simulink model "cascaded_droop_vi"  (R2021b)
settings: Solver=ode23t  StartTime=0.0  StopTime=20  RelTol=1e-3
values from neighbouring files (symbols this model uses):
  Cf_1 = 16e-6    (= 1.6e-05)    [parameters.m]
  fn = 50    [parameters.m]
  G_int = c2d(tf([wv 0],[1 wv]),Ts/2,'tustin')    [parameters.m]
  G_LPFd2 = c2d(tf([k*wn 0],[1 k*wn wn^2]),Ts/2,'tustin')    [parameters.m]
  Ilim = In    [parameters.m]
  ki_u = kp_u/Ti_u    [parameters.m]
  Kic_1 = (Rf_1)/T_i    (= 640)    [parameters.m]
  kp = delta_f/delta_P    (= 0.002)    [parameters.m]
  kp_u = Cf*w_c    [parameters.m]
  Kpc_1 = Rf_1/(exp(Rf_1/Lf_1*Ts/2)-1)    [parameters.m]
  Lf_1 = 5.6e-3    (= 0.0056)    [parameters.m]
  Lg_1 = 1e-3    (= 0.001)    [parameters.m]
  Lv = kQ/wn    [parameters.m]
  Pr = 2000    [parameters.m]
  RCf_1 = 0    [parameters.m]
  Rf_1 = 0.1    [parameters.m]
  Rg_1 = 0.08    [parameters.m]
  Rv = kQ/10    [parameters.m]
  Ts = 1/fs    (= 0.0003125)    [parameters.m]
  Ts_sim = Ts/100    (= 3.125e-06)    [parameters.m]
  Vdc = 800*sf_v    [parameters.m]
  Vn = 181*sqrt(2)*sf_v    [parameters.m]
  wn = 2*pi*fn    (= 314.159265359)    [parameters.m]
undefined symbols (not defined in the file or in its folder): DiscIntNeverNeededParam, plecs
libraries: spsVoltageMeasurementLib x15, spsCurrentMeasurementLib x12, spsabctoAlphaBetaZeroLib x10, spsThreePhaseSeriesRLCBranchLib x8, eeGeneralControl x7, spsThreePhaseVIMeasurementLib x4, spsGroundLib x3, spsThreePhaseSourceLib x2, spsDCVoltageSourceLib x2, spsEdgeDetectorLib x2, spsTriangleGeneratorLib x2, spsThreePhaseBreakerLib x2
(part 2 of 2)

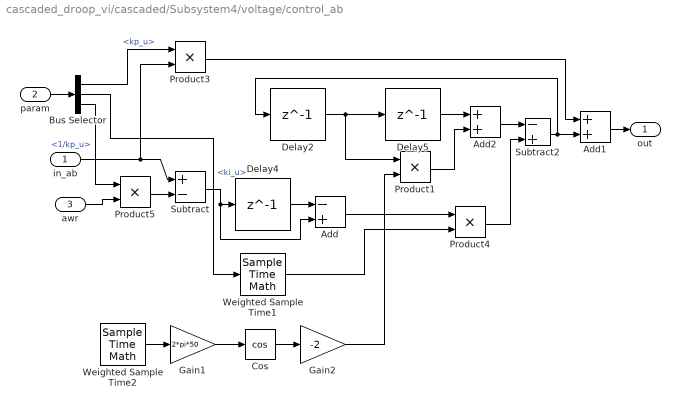
== system cascaded_droop_vi/cascaded/Subsystem4/voltage/control_ab ==
  in_ab : Inport
  param : Inport  Port=2
  awr : Inport  Port=3
  Add : Sum  Inputs=-+  AccumDataTypeStr=single
  Add1 : Sum
  Add2 : Sum
  Bus Selector : BusSelector  OutputSignals=kp_u,ki_u,1/kp_u
  Cos : Trigonometry  Operator=cos
  Delay2 : Delay  DelayLength=1  InitialCondition=0
  Delay4 : Delay  DelayLength=1  InitialCondition=0
  Delay5 : Delay  DelayLength=1  InitialCondition=0
  Gain1 : Gain  Gain=2*pi*50
  Gain2 : Gain  Gain=-2
  Product{1,3..5} (4 alike) : Product
  Subtract : Sum  Inputs=+-
  Subtract2 : Sum  Inputs=-+
  Weighted Sample Time1 : SampleTimeMath  TsampMathOp=*
  Weighted Sample Time2 : SampleTimeMath  TsampMathOp=Ts Only
  out : Outport  VectorParamsAs1DForOutWhenUnconnected=off
  wires:
  Gain2/1 -> Product1/2
  Cos/1 -> Gain2/1
  Gain1/1 -> Cos/1
  Weighted Sample Time2/1 -> Gain1/1
  Bus Selector/3 -> Product5/1  "<1/kp_u>"
  awr/1 -> Product5/2
  Product5/1 -> Subtract/2
  Weighted Sample Time1/1 -> Product4/2
  Bus Selector/2 -> Weighted Sample Time1/1  "<ki_u>"
  Bus Selector/1 -> Product3/1  "<kp_u>"
  Product3/1 -> Add1/1
  Add2/1 -> Subtract2/1
  Delay2/1 -> Delay5/1, Product1/1
  Subtract2/1 -> Add1/2, Delay2/1
  Delay5/1 -> Add2/1
  in_ab/1 -> Subtract/1, Product3/2
  Add/1 -> Product4/1
  Subtract/1 -> Add/2, Delay4/1
  Delay4/1 -> Add/1
  Product4/1 -> Subtract2/2
  Add1/1 -> out/1
  Product1/1 -> Add2/2
  param/1 -> Bus Selector/1

== system cascaded_droop_vi/cascaded/Subsystem4/voltage/current_FF ==
  a : Inport
  b : Inport  Port=2
  g_FF : Inport  Port=3
  Add5 : Sum
  Product : Product
  ab_out : Outport  VectorParamsAs1DForOutWhenUnconnected=off
  wires:
  Add5/1 -> ab_out/1
  a/1 -> Add5/1
  g_FF/1 -> Product/2
  b/1 -> Product/1
  Product/1 -> Add5/2

== system cascaded_droop_vi/cascaded controller/cascaded/Cascaded Loop/THI1 ==
  THI gain : Inport
  abc : Inport  Port=2
  ab : Inport  Port=3
  Add : Sum  Inputs=+++
  Add{1..4} (4 alike) : Sum
  Demux : Demux  Outputs=3
  Demux1 : Demux  Outputs=2
  Divide : Product  Inputs=*/*
  Fcn : Fcn  Expr=u^3
  Fcn1 : Fcn  Expr=u^3
  Fcn2 : Fcn  Expr=u^3
  Mux : Mux  Inputs=3
  Square : Math  Operator=square  SignedPower=on  RndMeth=Zero  SaturateOnIntegerOverflow=on
  Square1 : Math  Operator=square  SignedPower=on  RndMeth=Zero  SaturateOnIntegerOverflow=on
  abc_out : Outport  VectorParamsAs1DForOutWhenUnconnected=off
  wires:
  Demux/2 -> Add3/1, Fcn1/1
  Fcn2/1 -> Add/3
  Fcn1/1 -> Add/2
  Fcn/1 -> Add/1
  Mux/1 -> abc_out/1
  Add4/1 -> Mux/3
  Add2/1 -> Mux/1
  Add3/1 -> Mux/2
  Divide/1 -> Add4/2, Add3/2, Add2/2
  THI gain/1 -> Divide/3
  Add1/1 -> Divide/2
  Add/1 -> Divide/1
  Square1/1 -> Add1/2
  Square/1 -> Add1/1
  Demux1/2 -> Square1/1
  Demux1/1 -> Square/1
  ab/1 -> Demux1/1
  Demux/1 -> Fcn/1, Add2/1
  Demux/3 -> Add4/1, Fcn2/1
  abc/1 -> Demux/1

== system cascaded_droop_vi/cascaded controller/cascaded/Cascaded Loop/Virtual impedance ==
  Ig_ab : Inport
  Discrete Transfer Fcn2 : DiscreteTransferFcn  Numerator=G_int.num{1}  Denominator=G_int.den{1}
  Gain1 : Gain  Gain=Rv
  Gain2 : Gain  Gain=Lv
  Sum3 : Sum  Inputs=|++
  U_Lv_ab : Outport  VectorParamsAs1DForOutWhenUnconnected=off
  wires:
  Sum3/1 -> U_Lv_ab/1
  Gain1/1 -> Sum3/2
  Gain2/1 -> Sum3/1
  Ig_ab/1 -> Discrete Transfer Fcn2/1, Gain1/1
  Discrete Transfer Fcn2/1 -> Gain2/1

== system cascaded_droop_vi/cascaded controller/cascaded/Cascaded Loop/current ==
  param : Inport
  I_ab_ref : Inport  Port=2
  I_ab : Inport  Port=3
  U_ab : Inport  Port=4
  Udc : Inport  Port=5
  Bus Selector : BusSelector  OutputSignals=E1,g_ff_v
  Delay : Delay  DelayLength=1  InitialCondition=0
  Discrete Transfer Fcn : DiscreteTransferFcn  Numerator=G_LPFd2.num{1}  Denominator=G_LPFd2.den{1}
  Divide : Product  Inputs=*/
  Gain : Gain  Gain=1/2
  Subtract : Sum  Inputs=+-
  Subtract1 : Sum  Inputs=+-
  Voltage_lim : Subsystem
  control_ab : Subsystem
  voltage_FF : Subsystem
  U_ab_inv : Outport  VectorParamsAs1DForOutWhenUnconnected=off
  wires:
  Discrete Transfer Fcn/1 -> voltage_FF/2(b)
  voltage_FF/1(ab_out) -> Voltage_lim/1(ab_in), Subtract/1
  Delay/1 -> control_ab/3(awr)
  Gain/1 -> Divide/2
  Divide/1 -> U_ab_inv/1
  Udc/1 -> Voltage_lim/2(Vdc), Gain/1
  U_ab/1 -> Discrete Transfer Fcn/1
  Subtract/1 -> Delay/1
  Bus Selector/2 -> voltage_FF/3(g_FF)  "<g_ff_v>"
  I_ab/1 -> Subtract1/2
  Subtract1/1 -> control_ab/1(in_ab)
  control_ab/1(out) -> voltage_FF/1(a)
  param/1 -> control_ab/2(param), Bus Selector/1
  I_ab_ref/1 -> Subtract1/1
  Voltage_lim/1(ab_out) -> Subtract/2, Divide/1

== system cascaded_droop_vi/cascaded controller/cascaded/Cascaded Loop/voltage ==
  param : Inport
  U_ab_ref : Inport  Port=2
  U_ab : Inport  Port=3
  Ig_ab : Inport  Port=4
  Bus Selector : BusSelector  OutputSignals=g_ff_i,Isat
  Current_lim : Subsystem
  Delay : Delay  DelayLength=1  InitialCondition=0
  Subtract : Sum  Inputs=+-
  Subtract1 : Sum  Inputs=+-
  control_ab : Subsystem
  current_FF : Subsystem
  I_ab_ref : Outport  VectorParamsAs1DForOutWhenUnconnected=off
  wires:
  Bus Selector/2 -> Current_lim/2(Isat)  "<Isat>"
  U_ab_ref/1 -> Subtract1/1
  param/1 -> Bus Selector/1, control_ab/2(param)
  control_ab/1(out) -> current_FF/1(a)
  Subtract1/1 -> control_ab/1(in_ab)
  U_ab/1 -> Subtract1/2
  Bus Selector/1 -> current_FF/3(g_FF)  "<g_ff_i>"
  Subtract/1 -> Delay/1
  Ig_ab/1 -> current_FF/2(b)
  Current_lim/1(ab_out) -> I_ab_ref/1, Subtract/2
  Delay/1 -> control_ab/3(awr)
  current_FF/1(ab_out) -> Subtract/1, Current_lim/1(ab_in)

== system cascaded_droop_vi/cascaded controller/cascaded/power calculation grid side/abc to alpha-beta3 ==
  abc : Inport
  Demux : Demux  Outputs=3
  Terminator1 : Terminator
  abc to Alpha-Beta-Zero : spsabctoAlphaBetaZeroLib/abc to Alpha-Beta-Zero
  alpha : Outport
  beta : Outport  Port=2
  wires:
  abc to Alpha-Beta-Zero/1 -> Demux/1
  abc/1 -> abc to Alpha-Beta-Zero/1
  Demux/3 -> Terminator1/1
  Demux/2 -> beta/1
  Demux/1 -> alpha/1

== system cascaded_droop_vi/cascaded/Subsystem4/current/Voltage_lim/Subsystem ==
  a : Inport
  b : Inport  Port=2
  Relational Operator : RelationalOperator  Operator=>  OutDataTypeStr=boolean  RndMeth=Simplest
  Switch : Switch  Criteria=u2 > Threshold  Threshold=0.5
  max : Outport  VectorParamsAs1DForOutWhenUnconnected=off
  wires:
  a/1 -> Relational Operator/1, Switch/1
  Switch/1 -> max/1
  b/1 -> Relational Operator/2, Switch/3
  Relational Operator/1 -> Switch/2

== system cascaded_droop_vi/cascaded/Subsystem4/current/Voltage_lim/pythagoras ==
  ab : Inport
  Sqrt : Sqrt  SaturateOnIntegerOverflow=on
  Square : Math  Operator=square  SignedPower=on  RndMeth=Zero  SaturateOnIntegerOverflow=on
  Sum of Elements : Sum  Inputs=+
  |ab| : Outport  VectorParamsAs1DForOutWhenUnconnected=off
  wires:
  Sum of Elements/1 -> Sqrt/1
  ab/1 -> Square/1
  Square/1 -> Sum of Elements/1
  Sqrt/1 -> |ab|/1

== system cascaded_droop_vi/cascaded/Subsystem4/voltage/Current_lim/Subsystem ==
  a : Inport
  b : Inport  Port=2
  Relational Operator : RelationalOperator  Operator=>  OutDataTypeStr=boolean  RndMeth=Simplest
  Switch : Switch  Criteria=u2 > Threshold  Threshold=0.5
  max : Outport  VectorParamsAs1DForOutWhenUnconnected=off
  wires:
  Relational Operator/1 -> Switch/2
  b/1 -> Switch/3, Relational Operator/2
  Switch/1 -> max/1
  a/1 -> Switch/1, Relational Operator/1

== system cascaded_droop_vi/cascaded/Subsystem4/voltage/Current_lim/pythagoras ==
  ab : Inport
  Sqrt : Sqrt  SaturateOnIntegerOverflow=on
  Square : Math  Operator=square  SignedPower=on  RndMeth=Zero  SaturateOnIntegerOverflow=on
  Sum of Elements : Sum  Inputs=+
  |ab| : Outport  VectorParamsAs1DForOutWhenUnconnected=off
  wires:
  Sqrt/1 -> |ab|/1
  Square/1 -> Sum of Elements/1
  ab/1 -> Square/1
  Sum of Elements/1 -> Sqrt/1

== system cascaded_droop_vi/cascaded controller/cascaded/Cascaded Loop/current/Voltage_lim ==
  ab_in : Inport
  Vdc : Inport  Port=2
  Divide : Product  Inputs=*/
  Divide1 : Product  Inputs=**
  Gain : Gain  Gain=1/sqrt(3)
  Subsystem : Subsystem
  pythagoras : Subsystem
  ab_out : Outport  VectorParamsAs1DForOutWhenUnconnected=off
  wires:
  Gain/1 -> Divide/1, Subsystem/2(b)
  ab_in/1 -> Divide1/2, pythagoras/1(ab)
  pythagoras/1(|ab|) -> Subsystem/1(a)
  Vdc/1 -> Gain/1
  Subsystem/1(max) -> Divide/2
  Divide/1 -> Divide1/1
  Divide1/1 -> ab_out/1

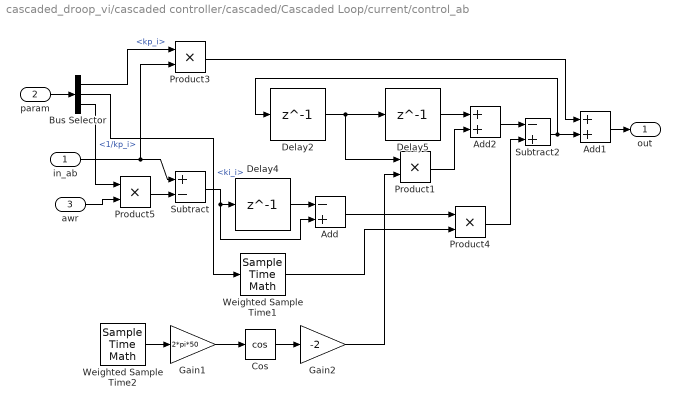
== system cascaded_droop_vi/cascaded controller/cascaded/Cascaded Loop/current/control_ab ==
  in_ab : Inport
  param : Inport  Port=2
  awr : Inport  Port=3
  Add : Sum  Inputs=-+  AccumDataTypeStr=single
  Add1 : Sum
  Add2 : Sum
  Bus Selector : BusSelector  OutputSignals=kp_i,ki_i,1/kp_i
  Cos : Trigonometry  Operator=cos
  Delay2 : Delay  DelayLength=1  InitialCondition=0
  Delay4 : Delay  DelayLength=1  InitialCondition=0
  Delay5 : Delay  DelayLength=1  InitialCondition=0
  Gain1 : Gain  Gain=2*pi*50
  Gain2 : Gain  Gain=-2
  Product{1,3..5} (4 alike) : Product
  Subtract : Sum  Inputs=+-
  Subtract2 : Sum  Inputs=-+
  Weighted Sample Time1 : SampleTimeMath  TsampMathOp=*
  Weighted Sample Time2 : SampleTimeMath  TsampMathOp=Ts Only
  out : Outport  VectorParamsAs1DForOutWhenUnconnected=off
  wires:
  param/1 -> Bus Selector/1
  Product1/1 -> Add2/2
  Add1/1 -> out/1
  Product4/1 -> Subtract2/2
  Delay4/1 -> Add/1
  Subtract/1 -> Delay4/1, Add/2
  Add/1 -> Product4/1
  in_ab/1 -> Product3/2, Subtract/1
  Delay5/1 -> Add2/1
  Subtract2/1 -> Delay2/1, Add1/2
  Delay2/1 -> Product1/1, Delay5/1
  Add2/1 -> Subtract2/1
  Product3/1 -> Add1/1
  Bus Selector/1 -> Product3/1  "<kp_i>"
  Bus Selector/2 -> Weighted Sample Time1/1  "<ki_i>"
  Weighted Sample Time1/1 -> Product4/2
  Product5/1 -> Subtract/2
  awr/1 -> Product5/2
  Bus Selector/3 -> Product5/1  "<1/kp_i>"
  Weighted Sample Time2/1 -> Gain1/1
  Gain1/1 -> Cos/1
  Cos/1 -> Gain2/1
  Gain2/1 -> Product1/2

== system cascaded_droop_vi/cascaded controller/cascaded/Cascaded Loop/current/voltage_FF ==
  a : Inport
  b : Inport  Port=2
  g_FF : Inport  Port=3
  Add5 : Sum
  Product : Product
  ab_out : Outport  VectorParamsAs1DForOutWhenUnconnected=off
  wires:
  Product/1 -> Add5/2
  b/1 -> Product/1
  g_FF/1 -> Product/2
  a/1 -> Add5/1
  Add5/1 -> ab_out/1

== system cascaded_droop_vi/cascaded controller/cascaded/Cascaded Loop/voltage/Current_lim ==
  ab_in : Inport
  Isat : Inport  Port=2
  Divide : Product  Inputs=*/
  Divide1 : Product  Inputs=**
  Subsystem : Subsystem
  pythagoras : Subsystem
  ab_out : Outport  VectorParamsAs1DForOutWhenUnconnected=off
  wires:
  Divide1/1 -> ab_out/1
  Divide/1 -> Divide1/1
  Subsystem/1(max) -> Divide/2
  pythagoras/1(|ab|) -> Subsystem/1(a)
  ab_in/1 -> pythagoras/1(ab), Divide1/2
  Isat/1 -> Subsystem/2(b), Divide/1

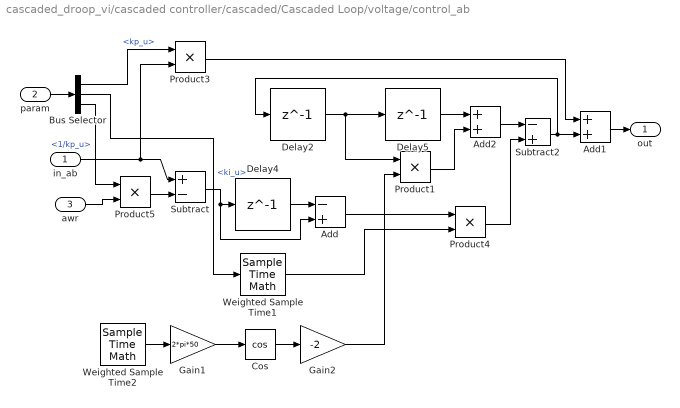
== system cascaded_droop_vi/cascaded controller/cascaded/Cascaded Loop/voltage/control_ab ==
  in_ab : Inport
  param : Inport  Port=2
  awr : Inport  Port=3
  Add : Sum  Inputs=-+  AccumDataTypeStr=single
  Add1 : Sum
  Add2 : Sum
  Bus Selector : BusSelector  OutputSignals=kp_u,ki_u,1/kp_u
  Cos : Trigonometry  Operator=cos
  Delay2 : Delay  DelayLength=1  InitialCondition=0
  Delay4 : Delay  DelayLength=1  InitialCondition=0
  Delay5 : Delay  DelayLength=1  InitialCondition=0
  Gain1 : Gain  Gain=2*pi*50
  Gain2 : Gain  Gain=-2
  Product{1,3..5} (4 alike) : Product
  Subtract : Sum  Inputs=+-
  Subtract2 : Sum  Inputs=-+
  Weighted Sample Time1 : SampleTimeMath  TsampMathOp=*
  Weighted Sample Time2 : SampleTimeMath  TsampMathOp=Ts Only
  out : Outport  VectorParamsAs1DForOutWhenUnconnected=off
  wires:
  Gain2/1 -> Product1/2
  Cos/1 -> Gain2/1
  Gain1/1 -> Cos/1
  Weighted Sample Time2/1 -> Gain1/1
  Bus Selector/3 -> Product5/1  "<1/kp_u>"
  awr/1 -> Product5/2
  Product5/1 -> Subtract/2
  Weighted Sample Time1/1 -> Product4/2
  Bus Selector/2 -> Weighted Sample Time1/1  "<ki_u>"
  Bus Selector/1 -> Product3/1  "<kp_u>"
  Product3/1 -> Add1/1
  Add2/1 -> Subtract2/1
  Delay2/1 -> Delay5/1, Product1/1
  Subtract2/1 -> Add1/2, Delay2/1
  Delay5/1 -> Add2/1
  in_ab/1 -> Subtract/1, Product3/2
  Add/1 -> Product4/1
  Subtract/1 -> Add/2, Delay4/1
  Delay4/1 -> Add/1
  Product4/1 -> Subtract2/2
  Add1/1 -> out/1
  Product1/1 -> Add2/2
  param/1 -> Bus Selector/1

== system cascaded_droop_vi/cascaded controller/cascaded/Cascaded Loop/voltage/current_FF ==
  a : Inport
  b : Inport  Port=2
  g_FF : Inport  Port=3
  Add5 : Sum
  Product : Product
  ab_out : Outport  VectorParamsAs1DForOutWhenUnconnected=off
  wires:
  Add5/1 -> ab_out/1
  a/1 -> Add5/1
  g_FF/1 -> Product/2
  b/1 -> Product/1
  Product/1 -> Add5/2

== system cascaded_droop_vi/cascaded controller/cascaded/Cascaded Loop/current/Voltage_lim/Subsystem ==
  a : Inport
  b : Inport  Port=2
  Relational Operator : RelationalOperator  Operator=>  OutDataTypeStr=boolean  RndMeth=Simplest
  Switch : Switch  Criteria=u2 > Threshold  Threshold=0.5
  max : Outport  VectorParamsAs1DForOutWhenUnconnected=off
  wires:
  a/1 -> Relational Operator/1, Switch/1
  Switch/1 -> max/1
  b/1 -> Relational Operator/2, Switch/3
  Relational Operator/1 -> Switch/2

== system cascaded_droop_vi/cascaded controller/cascaded/Cascaded Loop/current/Voltage_lim/pythagoras ==
  ab : Inport
  Sqrt : Sqrt  SaturateOnIntegerOverflow=on
  Square : Math  Operator=square  SignedPower=on  RndMeth=Zero  SaturateOnIntegerOverflow=on
  Sum of Elements : Sum  Inputs=+
  |ab| : Outport  VectorParamsAs1DForOutWhenUnconnected=off
  wires:
  Sum of Elements/1 -> Sqrt/1
  ab/1 -> Square/1
  Square/1 -> Sum of Elements/1
  Sqrt/1 -> |ab|/1

== system cascaded_droop_vi/cascaded controller/cascaded/Cascaded Loop/voltage/Current_lim/Subsystem ==
  a : Inport
  b : Inport  Port=2
  Relational Operator : RelationalOperator  Operator=>  OutDataTypeStr=boolean  RndMeth=Simplest
  Switch : Switch  Criteria=u2 > Threshold  Threshold=0.5
  max : Outport  VectorParamsAs1DForOutWhenUnconnected=off
  wires:
  Relational Operator/1 -> Switch/2
  b/1 -> Switch/3, Relational Operator/2
  Switch/1 -> max/1
  a/1 -> Switch/1, Relational Operator/1

== system cascaded_droop_vi/cascaded controller/cascaded/Cascaded Loop/voltage/Current_lim/pythagoras ==
  ab : Inport
  Sqrt : Sqrt  SaturateOnIntegerOverflow=on
  Square : Math  Operator=square  SignedPower=on  RndMeth=Zero  SaturateOnIntegerOverflow=on
  Sum of Elements : Sum  Inputs=+
  |ab| : Outport  VectorParamsAs1DForOutWhenUnconnected=off
  wires:
  Sqrt/1 -> |ab|/1
  Square/1 -> Sum of Elements/1
  ab/1 -> Square/1
  Sum of Elements/1 -> Sqrt/1
